simulink model "Open_Jackson_Network"  (Simulink 7.9)
settings: Solver=VariableStepDiscrete  StartTime=0.0  StopTime=50  RelTol=1e-3
undefined symbols (not defined in the file or in its folder): des, gcbh
libraries: simeventslib x7
settings Model: Creator=tsprock3  LastModifiedBy=tsprock3
settings DebuggingCC: SolverPrmCheckMsg=none  SimStateOlderReleaseMsg=warning

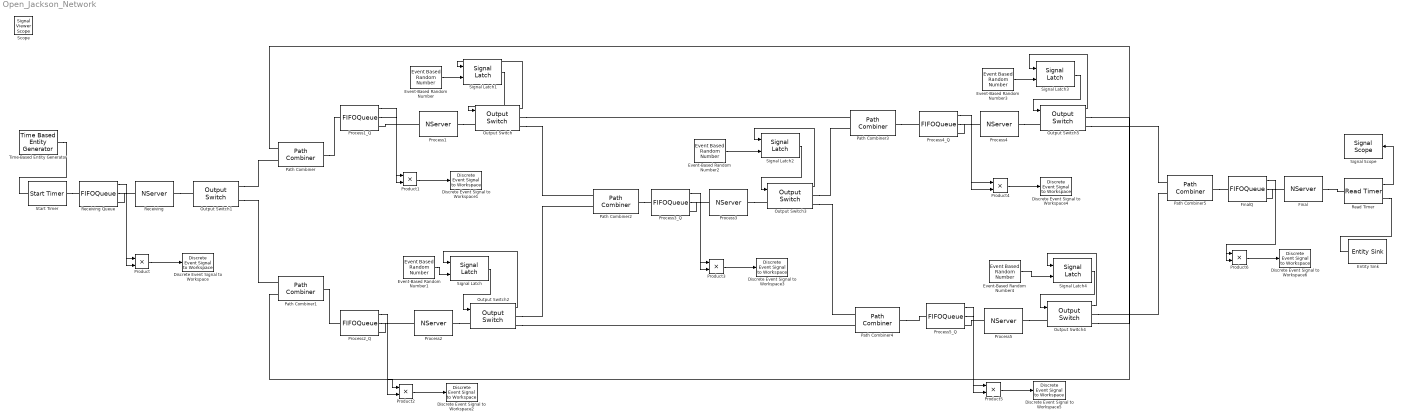
== system Open_Jackson_Network ==
  Discrete Event Signal to Workspace : simeventslib/SimEvents Sinks/Discrete Event Signal to Workspace  VariableName=Receiving_Metric  SaveFormat=Structure With Time  isMonitorOnly=off  isRecordIC=off
  Discrete Event Signal to Workspace1 : simeventslib/SimEvents Sinks/Discrete Event Signal to Workspace  VariableName=Q1_Metric  SaveFormat=Structure With Time  isMonitorOnly=off  isRecordIC=off
  Discrete Event Signal to Workspace2 : simeventslib/SimEvents Sinks/Discrete Event Signal to Workspace  VariableName=Q2_Metric  SaveFormat=Structure With Time  isMonitorOnly=off  isRecordIC=off
  Discrete Event Signal to Workspace3 : simeventslib/SimEvents Sinks/Discrete Event Signal to Workspace  VariableName=Q3_Metric  SaveFormat=Structure With Time  isMonitorOnly=off  isRecordIC=off
  Discrete Event Signal to Workspace4 : simeventslib/SimEvents Sinks/Discrete Event Signal to Workspace  VariableName=Q4_Metric  SaveFormat=Structure With Time  isMonitorOnly=off  isRecordIC=off
  Discrete Event Signal to Workspace5 : simeventslib/SimEvents Sinks/Discrete Event Signal to Workspace  VariableName=Q5_Metric  SaveFormat=Structure With Time  isMonitorOnly=off  isRecordIC=off
  Discrete Event Signal to Workspace6 : simeventslib/SimEvents Sinks/Discrete Event Signal to Workspace  VariableName=Final_Metric  SaveFormat=Structure With Time  isMonitorOnly=off  isRecordIC=off
  Entity Sink : EntitySink
  Event-Based Random Number : EventBasedRandomNumber  Distribution=Arbitrary discrete  valueVecCont=[1 2]  cdfVecCont=[.25 .75]  valueVecDisc=[1 2]  probVecDisc=[0.25 0.75]  Seed=17144
  Event-Based Random Number1 : EventBasedRandomNumber  Distribution=Arbitrary discrete  valueVecCont=[1 2]  cdfVecCont=[.25 .75]  valueVecDisc=[1 2]  probVecDisc=[0.25 0.75]  Seed=20361
  Event-Based Random Number2 : EventBasedRandomNumber  Distribution=Arbitrary discrete  valueVecCont=[1 2]  cdfVecCont=[.25 .75]  valueVecDisc=[1 2]  probVecDisc=[0.25 0.75]  Seed=23578
  Event-Based Random Number3 : EventBasedRandomNumber  Distribution=Arbitrary discrete  valueVecCont=[1 2]  cdfVecCont=[.25 .75]  valueVecDisc=[1 2]  probVecDisc=[0.1 0.9]  Seed=26795
  Event-Based Random Number4 : EventBasedRandomNumber  Distribution=Arbitrary discrete  valueVecCont=[1 2]  cdfVecCont=[.25 .75]  valueVecDisc=[1 2]  probVecDisc=[0.9 0.1]  Seed=30012
  Final : NServer
  FinalQ : FIFOQueue  Capacity=inf  StatAverageWait=on  StatAverageQueueLength=on
      settings: OutputPortMap=o2,o3
  Output Switch{,2..5} (5 alike) : OutputSwitch  NumberOutputPorts=2  SwitchingCriterion=From signal port p  StatNumberDeparted=on
  Output Switch1 : OutputSwitch  NumberOutputPorts=2
  Path Combiner{,1..5} (6 alike) : PathCombiner  NumberInputPorts=2
  Process1 : NServer  NumberOfServers=4  ServiceTime=3
  Process1_Q : FIFOQueue  Capacity=inf  StatAverageWait=on  StatAverageQueueLength=on
      settings: OutputPortMap=o2,o3
  Process2 : NServer  NumberOfServers=1  ServiceTime=3
  Process2_Q : FIFOQueue  Capacity=inf  StatAverageWait=on  StatAverageQueueLength=on
      settings: OutputPortMap=o2,o3
  Process3 : NServer  NumberOfServers=2  ServiceTime=2
  Process3_Q : FIFOQueue  Capacity=inf  StatAverageWait=on  StatAverageQueueLength=on
      settings: OutputPortMap=o2,o3
  Process4 : NServer  NumberOfServers=3  ServiceTime=5
  Process4_Q : FIFOQueue  Capacity=inf  StatAverageWait=on  StatAverageQueueLength=on
      settings: OutputPortMap=o2,o3
  Process5 : NServer  ServiceTime=5
  Process5_Q : FIFOQueue  Capacity=inf  StatAverageWait=on  StatAverageQueueLength=on
      settings: OutputPortMap=o2,o3
  Product{,1..6} (7 alike) : Product  RndMeth=Zero
  Read Timer : ReadTimer  StatAverageTimeElapsed=on
      settings: OutputPortMap=o3
  Receiving : NServer  NumberOfServers=3
  Receiving Queue : FIFOQueue  Capacity=inf  StatAverageWait=on  StatAverageQueueLength=on
      settings: OutputPortMap=o2,o3
  Signal Latch{,1..4} (5 alike) : SignalLatch  InitialMemoryValue=1  ReadMemoryUpon=Write to memory event
      settings: InputPortMap=u0,u2  OutputPortMap=o2
  Signal Scope : SignalScope  LoadFcn=des.scope.CallbackSupport('seLoadFcn',gcbh)  StartFcn=des.scope.CallbackSupport('seStartFcn',gcbh)  StopFcn=des.scope.CallbackSupport('seStopFcn',gcbh)
      settings: CopyFcn=des.scope.CallbackSupport('seCopyFcn',gcbh)  DeleteFcn=des.scope.CallbackSupport('seDeleteFcn',gcbh)  PreSaveFcn=des.scope.CallbackSupport('sePreSaveFcn',gcbh)  NameChangeFcn=des.scope.CallbackSupport('seNameChangeFcn',gcbh)  OpenFcn=des.scope.CallbackSupport('seOpenFcn',gcbh)
  Start Timer : StartTimer
  Time-Based Entity Generator : TimeBasedEntityGenerator  Distribution=Exponential  InitialSeed=33229
  Scope : SignalViewerScope  IOType=viewer  RefreshTime=0.035000
  wires:
  Event-Based Random Number2/1 -> Signal Latch2/2
  Event-Based Random Number4/1 -> Signal Latch4/2
  Event-Based Random Number1/1 -> Signal Latch/2
  Signal Latch/1 -> Output Switch2/1
  Output Switch2/1 -> Signal Latch/1
  Event-Based Random Number/1 -> Signal Latch1/2
  Output Switch/1 -> Signal Latch1/1
  Signal Latch1/1 -> Output Switch/1
  Output Switch3/1 -> Signal Latch2/1
  Signal Latch2/1 -> Output Switch3/1
  Signal Latch4/1 -> Output Switch4/1
  Output Switch4/1 -> Signal Latch4/1
  Output Switch5/1 -> Signal Latch3/1
  Signal Latch3/1 -> Output Switch5/1
  Event-Based Random Number3/1 -> Signal Latch3/2
  Process5_Q/1 -> Product5/1
  Process5_Q/2 -> Product5/2
  Product5/1 -> Discrete Event Signal to Workspace5/1
  Product/1 -> Discrete Event Signal to Workspace/1
  Receiving Queue/1 -> Product/1
  Receiving Queue/2 -> Product/2
  Product2/1 -> Discrete Event Signal to Workspace2/1
  Process2_Q/2 -> Product2/2
  Process2_Q/1 -> Product2/1
  Product1/1 -> Discrete Event Signal to Workspace1/1
  Process1_Q/2 -> Product1/2
  Process1_Q/1 -> Product1/1
  Product3/1 -> Discrete Event Signal to Workspace3/1
  Process3_Q/2 -> Product3/2
  Process3_Q/1 -> Product3/1
  Product4/1 -> Discrete Event Signal to Workspace4/1
  Process4_Q/2 -> Product4/2
  Process4_Q/1 -> Product4/1
  Product6/1 -> Discrete Event Signal to Workspace6/1
  FinalQ/2 -> Product6/2
  FinalQ/1 -> Product6/1
  Read Timer/1 -> Signal Scope/1
  connections:
  Process1_Q/RConn1 -- Process1/LConn1
  Process2_Q/RConn1 -- Process2/LConn1
  Process3_Q/RConn1 -- Process3/LConn1
  Process4_Q/RConn1 -- Process4/LConn1
  Process5_Q/RConn1 -- Process5/LConn1
  Path Combiner/RConn1 -- Process1_Q/LConn1
  Receiving Queue/RConn1 -- Receiving/LConn1
  Receiving/RConn1 -- Output Switch1/LConn1
  Output Switch1/RConn1 -- Path Combiner/LConn2
  Output Switch1/RConn2 -- Path Combiner1/LConn1
  Path Combiner1/RConn1 -- Process2_Q/LConn1
  Output Switch/RConn2 -- Path Combiner2/LConn1
  Process1/RConn1 -- Output Switch/LConn1
  Process2/RConn1 -- Output Switch2/LConn1
  Output Switch2/RConn1 -- Path Combiner2/LConn2
  Path Combiner3/RConn1 -- Process4_Q/LConn1
  Path Combiner4/RConn1 -- Process5_Q/LConn1
  Output Switch2/RConn2 -- Path Combiner4/LConn2
  Output Switch/RConn1 -- Path Combiner3/LConn1
  Process3/RConn1 -- Output Switch3/LConn1
  Output Switch3/RConn1 -- Path Combiner3/LConn2
  Output Switch3/RConn2 -- Path Combiner4/LConn1
  Process5/RConn1 -- Output Switch4/LConn1
  Process4/RConn1 -- Output Switch5/LConn1
  Output Switch5/RConn1 -- Path Combiner1/LConn2
  Output Switch4/RConn2 -- Path Combiner/LConn1
  FinalQ/RConn1 -- Final/LConn1
  Output Switch5/RConn2 -- Path Combiner5/LConn1
  Output Switch4/RConn1 -- Path Combiner5/LConn2
  Path Combiner2/RConn1 -- Process3_Q/LConn1
  Start Timer/RConn1 -- Receiving Queue/LConn1
  Time-Based Entity Generator/RConn1 -- Start Timer/LConn1
  Final/RConn1 -- Read Timer/LConn1
  Read Timer/RConn1 -- Entity Sink/LConn1
  Path Combiner5/RConn1 -- FinalQ/LConn1
